simulink model "sys"  (R2024a)
settings: Solver=ode4  StartTime=0.0  StopTime=20  RelTol=1e-3
values from neighbouring files (symbols this model uses):
  d = 0.3    [params.m]
settings Model: Creator=truong giang  LastModifiedBy=TRUONG GIANG
settings SolverCC: AlgebraicLoopSolver=TrustRegion
settings DataIOCC: ReturnWorkspaceOutputs=off
settings OptimizationCC: LifeSpan=inf
settings DebuggingCC: UnconnectedInputMsg=warning  UnconnectedOutputMsg=warning  UnconnectedLineMsg=warning  ArithmeticOperatorsInVariantConditions=warning
settings ModelReferenceCC: EnableRefExpFcnMdlSchedulingChecks=on
settings SFSimCC: SimUseLocalCustomCode=off  CustomCodeUndefinedFunction=UseInterfaceOnly
settings RTWCC: RTWUseLocalCustomCode=off  GPUComputeCapability=3.5
settings CodeAppCC: StateflowObjectComments=on

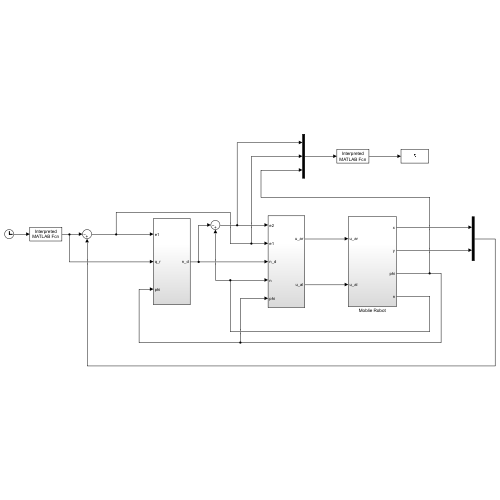
[thumbnail: Simulink's stored preview of the top-level diagram]
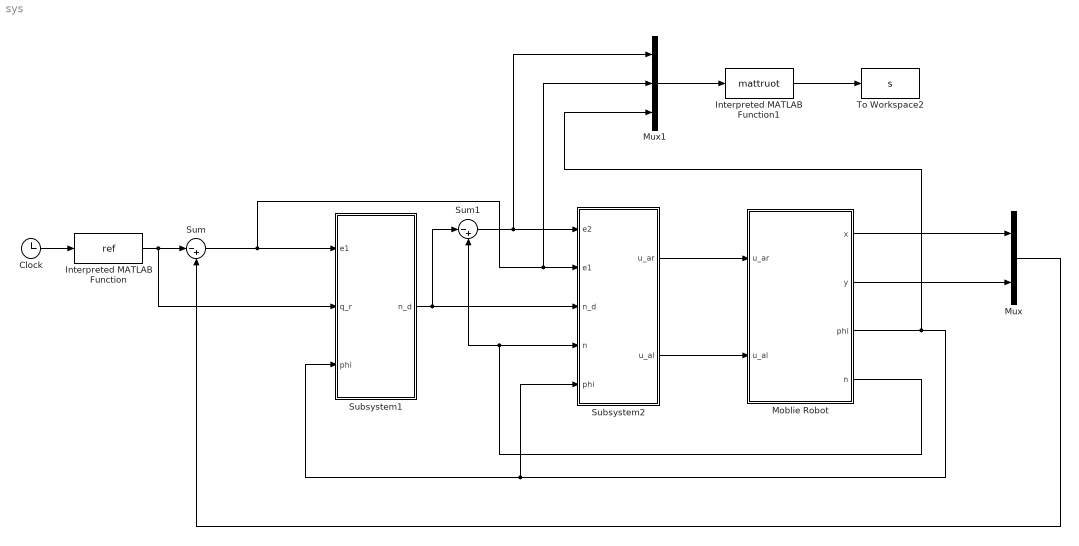
== system sys ==
  Clock : Clock
  Interpreted MATLAB Function : MATLABFcn  MATLABFcn=ref  OutputDimensions=2
  Interpreted MATLAB Function1 : MATLABFcn  MATLABFcn=mattruot  OutputDimensions=2
  Moblie Robot : Subsystem
  Mux : Mux  Inputs=2
  Mux1 : Mux  Inputs=3
  Subsystem1 : Subsystem
  Subsystem2 : Subsystem
  Sum : Sum  Inputs=|-+
  Sum1 : Sum  Inputs=|-+
  To Workspace2 : ToWorkspace  VariableName=s  SampleTime=0.02
  wires:
  Clock/1 -> Interpreted MATLAB Function/1
  Subsystem1/1(n_d) -> Sum1/1, Subsystem2/3(n_d)
  Subsystem2/2(u_al) -> Moblie Robot/2(u_al)
  Subsystem2/1(u_ar) -> Moblie Robot/1(u_ar)
  Moblie Robot/4(n) -> Sum1/2, Subsystem2/4(n)
  Moblie Robot/3(phi) -> Mux1/3, Subsystem2/5(phi), Subsystem1/3(phi)
  Moblie Robot/2(y) -> Mux/2
  Moblie Robot/1(x) -> Mux/1
  Mux/1 -> Sum/2
  Interpreted MATLAB Function/1 -> Subsystem1/2(q_r), Sum/1
  Sum/1 -> Mux1/2, Subsystem2/2(e1), Subsystem1/1(e1)
  Sum1/1 -> Mux1/1, Subsystem2/1(e2)
  Mux1/1 -> Interpreted MATLAB Function1/1
  Interpreted MATLAB Function1/1 -> To Workspace2/1

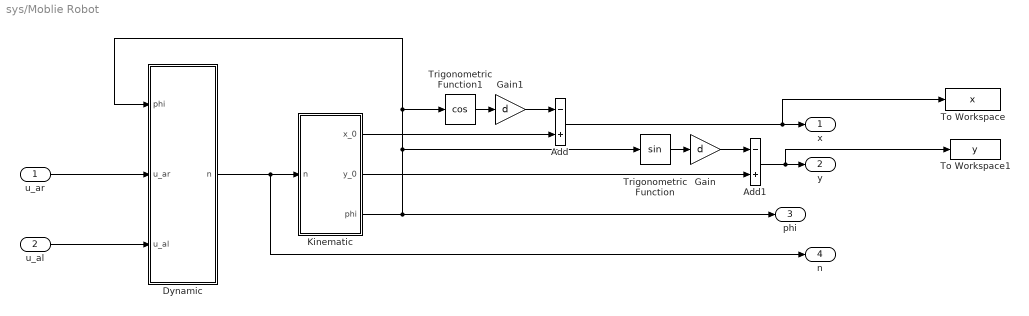
== system sys/Moblie Robot ==
  u_ar : Inport
  u_al : Inport  Port=2
  Add : Sum  Inputs=-+
  Add1 : Sum  Inputs=-+
  Dynamic : Subsystem
  Gain : Gain  Gain=d
  Gain1 : Gain  Gain=d
  Kinematic : Subsystem
  To Workspace : ToWorkspace  VariableName=x  SampleTime=0.02
      settings: Save2DSignal=2-D array (concatenate along first dimension)
  To Workspace1 : ToWorkspace  VariableName=y  SampleTime=0.02
      settings: Save2DSignal=2-D array (concatenate along first dimension)
  Trigonometric Function : Trigonometry
  Trigonometric Function1 : Trigonometry  Operator=cos
  x : Outport
  y : Outport  Port=2
  phi : Outport  Port=3
  n : Outport  Port=4
  wires:
  Kinematic/3(phi) -> Trigonometric Function/1, Trigonometric Function1/1, Dynamic/1(phi), phi/1
  u_ar/1 -> Dynamic/2(u_ar)
  u_al/1 -> Dynamic/3(u_al)
  Trigonometric Function1/1 -> Gain1/1
  Gain1/1 -> Add/1
  Kinematic/1(x_0) -> Add/2
  Add/1 -> To Workspace/1, x/1
  Kinematic/2(y_0) -> Add1/2
  Gain/1 -> Add1/1
  Trigonometric Function/1 -> Gain/1
  Add1/1 -> To Workspace1/1, y/1
  Dynamic/1(n) -> n/1, Kinematic/1(n)

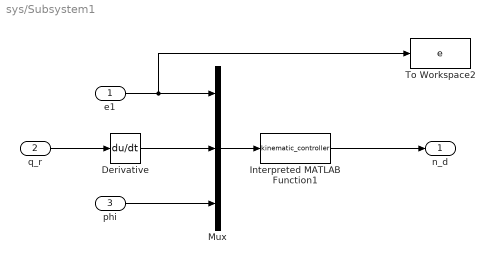
== system sys/Subsystem1 ==
  e1 : Inport
  q_r : Inport  Port=2
  phi : Inport  Port=3
  Derivative : Derivative
  Interpreted MATLAB Function1 : MATLABFcn  MATLABFcn=kinematic_controller  OutputDimensions=2
  Mux : Mux  Inputs=3
  To Workspace2 : ToWorkspace  VariableName=e  SampleTime=0.02
  n_d : Outport
  wires:
  Mux/1 -> Interpreted MATLAB Function1/1
  phi/1 -> Mux/3
  e1/1 -> To Workspace2/1, Mux/1
  Interpreted MATLAB Function1/1 -> n_d/1
  Derivative/1 -> Mux/2
  q_r/1 -> Derivative/1

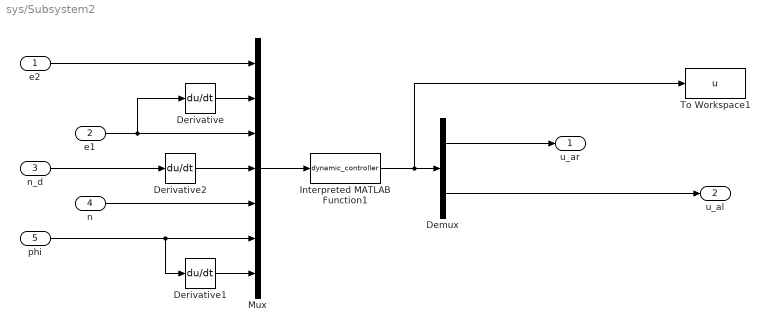
== system sys/Subsystem2 ==
  e2 : Inport
  e1 : Inport  Port=2
  n_d : Inport  Port=3
  n : Inport  Port=4
  phi : Inport  Port=5
  Demux : Demux  Outputs=2
  Derivative : Derivative
  Derivative1 : Derivative
  Derivative2 : Derivative
  Interpreted MATLAB Function1 : MATLABFcn  MATLABFcn=dynamic_controller  OutputDimensions=2
  Mux : Mux  Inputs=7
  To Workspace1 : ToWorkspace  VariableName=u  SampleTime=0.02
      settings: Decimation=2  Save2DSignal=2-D array (concatenate along first dimension)
  u_ar : Outport
  u_al : Outport  Port=2
  wires:
  phi/1 -> Derivative1/1, Mux/6
  n/1 -> Mux/5
  Derivative/1 -> Mux/2
  e2/1 -> Mux/1
  Mux/1 -> Interpreted MATLAB Function1/1
  Derivative1/1 -> Mux/7
  Demux/1 -> u_ar/1
  Interpreted MATLAB Function1/1 -> To Workspace1/1, Demux/1
  Demux/2 -> u_al/1
  e1/1 -> Derivative/1, Mux/3
  Derivative2/1 -> Mux/4
  n_d/1 -> Derivative2/1

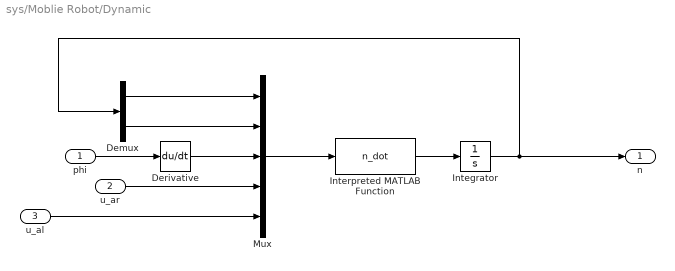
== system sys/Moblie Robot/Dynamic ==
  phi : Inport
  u_ar : Inport  Port=2
  u_al : Inport  Port=3
  Demux : Demux  Outputs=2
  Derivative : Derivative
  Integrator : Integrator
  Interpreted MATLAB Function : MATLABFcn  MATLABFcn=n_dot  OutputDimensions=2
  Mux : Mux  Inputs=5
  n : Outport
  wires:
  Interpreted MATLAB Function/1 -> Integrator/1
  Mux/1 -> Interpreted MATLAB Function/1
  Demux/1 -> Mux/1
  Demux/2 -> Mux/2
  Derivative/1 -> Mux/3
  phi/1 -> Derivative/1
  u_ar/1 -> Mux/4
  u_al/1 -> Mux/5
  Integrator/1 -> Demux/1, n/1

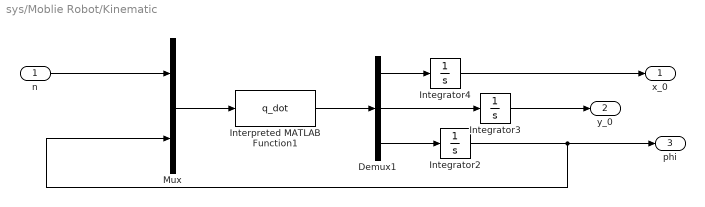
== system sys/Moblie Robot/Kinematic ==
  n : Inport
  Demux1 : Demux  Outputs=3
  Integrator2 : Integrator  InitialCondition=0.0
  Integrator3 : Integrator  InitialCondition=0.0
  Integrator4 : Integrator  InitialCondition=0.0
  Interpreted MATLAB Function1 : MATLABFcn  MATLABFcn=q_dot  OutputDimensions=3
  Mux : Mux  Inputs=2
  x_0 : Outport
  y_0 : Outport  Port=2
  phi : Outport  Port=3
  wires:
  Mux/1 -> Interpreted MATLAB Function1/1
  n/1 -> Mux/1
  Interpreted MATLAB Function1/1 -> Demux1/1
  Integrator4/1 -> x_0/1
  Demux1/1 -> Integrator4/1
  Integrator3/1 -> y_0/1
  Demux1/2 -> Integrator3/1
  Integrator2/1 -> Mux/2, phi/1
  Demux1/3 -> Integrator2/1
